simulink model "PMSM_NFLUX_v1_1"  (R2023b)
settings: Solver=FixedStepDiscrete  StartTime=0.0  StopTime=50  FixedStep=0.0001  RelTol=1e-3
values from neighbouring files (symbols this model uses):
  B = 8.0E-5    [PMSM_NFLUX.sldd]    (also in PMSM_NFLUX_backup_before_Simulink_RsStandstillID_20260617_154804.sldd; init_PMSM_NFLUX.m = single(8e-5))
  curr_d_ki = 35.0    [PMSM_NFLUX.sldd]    (also in PMSM_NFLUX_backup_before_Simulink_RsStandstillID_20260617_154804.sldd; init_PMSM_NFLUX.m = 35)
  curr_d_kp = 0.017    [PMSM_NFLUX.sldd]    (also in PMSM_NFLUX_backup_before_Simulink_RsStandstillID_20260617_154804.sldd; init_PMSM_NFLUX.m = 0.017)
  curr_q_ki = 35.0    [PMSM_NFLUX.sldd]    (also in PMSM_NFLUX_backup_before_Simulink_RsStandstillID_20260617_154804.sldd; init_PMSM_NFLUX.m = 35)
  curr_q_kp = 0.017    [PMSM_NFLUX.sldd]    (also in PMSM_NFLUX_backup_before_Simulink_RsStandstillID_20260617_154804.sldd; init_PMSM_NFLUX.m = 0.017)
  flux = 0.016884    [PMSM_NFLUX.sldd]    (also in PMSM_NFLUX_backup_before_Simulink_RsStandstillID_20260617_154804.sldd; init_PMSM_NFLUX.m = single(0.016884))
  Gamma = 100000.0    [PMSM_NFLUX.sldd]    (also in PMSM_NFLUX_backup_before_Simulink_RsStandstillID_20260617_154804.sldd; init_PMSM_NFLUX.m = single(100000.0))
  iq_handover = 0.4    [PMSM_NFLUX.sldd]    (also in PMSM_NFLUX_backup_before_Simulink_RsStandstillID_20260617_154804.sldd; init_PMSM_NFLUX.m = single(0.4))
  iq_ref_slew_down = 2.0    [PMSM_NFLUX.sldd]    (also in PMSM_NFLUX_backup_before_Simulink_RsStandstillID_20260617_154804.sldd; init_PMSM_NFLUX.m = single(2.0))
  iq_ref_slew_up = 5.0    [PMSM_NFLUX.sldd]    (also in PMSM_NFLUX_backup_before_Simulink_RsStandstillID_20260617_154804.sldd; init_PMSM_NFLUX.m = single(5.0))
  J = 7.5E-5    [PMSM_NFLUX.sldd]    (also in PMSM_NFLUX_backup_before_Simulink_RsStandstillID_20260617_154804.sldd; init_PMSM_NFLUX.m = single(75e-6))
  L = 0.00535    [PMSM_NFLUX.sldd]    (also in PMSM_NFLUX_backup_before_Simulink_RsStandstillID_20260617_154804.sldd; init_PMSM_NFLUX.m = single(0.00535))
  load_torque = 0.0    [PMSM_NFLUX.sldd]    (also in PMSM_NFLUX_backup_before_Simulink_RsStandstillID_20260617_154804.sldd; init_PMSM_NFLUX.m = single(0.0))
  LPF_K = 0.003    [PMSM_NFLUX.sldd]    (also in PMSM_NFLUX_backup_before_Simulink_RsStandstillID_20260617_154804.sldd; init_PMSM_NFLUX.m = single(0.003))
  PLL_Ki = 2500.0    [PMSM_NFLUX.sldd]    (also in PMSM_NFLUX_backup_before_Simulink_RsStandstillID_20260617_154804.sldd; init_PMSM_NFLUX.m = single(2500))
  PLL_Kp = 212.1    [PMSM_NFLUX.sldd]    (also in PMSM_NFLUX_backup_before_Simulink_RsStandstillID_20260617_154804.sldd; init_PMSM_NFLUX.m = single(212.1))
  PLL_OmegaLimit = 6283.18555    [PMSM_NFLUX.sldd]    (also in PMSM_NFLUX_backup_before_Simulink_RsStandstillID_20260617_154804.sldd; init_PMSM_NFLUX.m = single(2.0 * pi * 1000.0))
  Pn = 4.0    [PMSM_NFLUX.sldd]    (also in PMSM_NFLUX_backup_before_Simulink_RsStandstillID_20260617_154804.sldd; init_PMSM_NFLUX.m = single(4))
  PWM_HalfPeriod = 8000.0    [PMSM_NFLUX.sldd]    (also in PMSM_NFLUX_backup_before_Simulink_RsStandstillID_20260617_154804.sldd; init_PMSM_NFLUX.m = single(8000))
  Rs = 6.97    [PMSM_NFLUX.sldd]    (also in PMSM_NFLUX_backup_before_Simulink_RsStandstillID_20260617_154804.sldd; init_PMSM_NFLUX.m = single(6.97))
  spd_ki = 0.00165394868    [PMSM_NFLUX.sldd]    (also in PMSM_NFLUX_backup_before_Simulink_RsStandstillID_20260617_154804.sldd; init_PMSM_NFLUX.m = (B * speed_bw / Kt) * rpm_to_radps)
  spd_kp = 0.001550577    [PMSM_NFLUX.sldd]    (also in PMSM_NFLUX_backup_before_Simulink_RsStandstillID_20260617_154804.sldd; init_PMSM_NFLUX.m = (J * speed_bw / Kt) * rpm_to_radps)
  theta_handover_slew_limit = 5.0    [PMSM_NFLUX.sldd]    (also in PMSM_NFLUX_backup_before_Simulink_RsStandstillID_20260617_154804.sldd; init_PMSM_NFLUX.m = single(5.0))
  Tpwm = 16000.0    [PMSM_NFLUX.sldd]    (also in PMSM_NFLUX_backup_before_Simulink_RsStandstillID_20260617_154804.sldd; init_PMSM_NFLUX.m = 2 * PWM_HalfPeriod)
  Ts = 0.0001    [PMSM_NFLUX.sldd]    (also in PMSM_NFLUX_backup_before_Simulink_RsStandstillID_20260617_154804.sldd; init_PMSM_NFLUX.m = 0.0001)
  Udc = 24.0    [PMSM_NFLUX.sldd]    (also in PMSM_NFLUX_backup_before_Simulink_RsStandstillID_20260617_154804.sldd; init_PMSM_NFLUX.m = single(24.0))
undefined symbols (not defined in the file or in its folder): DiscIntNeverNeededParam, magnitude, sigbuilder_block
libraries: slpidlib x4, mcbplantlib x1, simulink x1, autolibpmsmexterior x1
(part 2 of 2)

== system PMSM_NFLUX_v1_1/FOC/current_loop/SVPWM/ei_t ==
  Vabc : Inport  OutDataTypeStr=single
  Demux : Demux  Outputs=3
  Gain : Gain  Gain=-1/2  OutDataTypeStr=single
  Min : MinMax  Inputs=3  OutDataTypeStr=single
  Min1 : MinMax  Function=max  Inputs=3  OutDataTypeStr=single
  Sum : Sum  Inputs=|++  OutDataTypeStr=single
  ei_t : Outport  OutDataTypeStr=single
  wires:
  Min/1 -> Sum/1
  Sum/1 -> Gain/1
  Min1/1 -> Sum/2
  Gain/1 -> ei_t/1
  Vabc/1 -> Demux/1
  Demux/1 -> Min1/1, Min/1
  Demux/2 -> Min/2, Min1/2
  Demux/3 -> Min1/3, Min/3

== system PMSM_NFLUX_v1_1/FOC/current_loop/Subsystem/If Action Subsystem ==
  Action Port : ActionPort  ActionPortLabel=case [ 1 ]:
  Constant : Constant  Value=0  OutDataTypeStr=single
  Constant1 : Constant  Value=0  OutDataTypeStr=single
  theta_fd : Outport
  iq_ref : Outport  Port=2
  wires:
  Constant/1 -> theta_fd/1
  Constant1/1 -> iq_ref/1

== system PMSM_NFLUX_v1_1/FOC/current_loop/Subsystem/If Action Subsystem1 ==
  Action Port : ActionPort  ActionPortLabel=case [ 2 ]:
  Constant : Constant  Value=0  OutDataTypeStr=single
  Constant1 : Constant  OutDataTypeStr=single
  theta_fd : Outport
  iq_ref : Outport  Port=2
  wires:
  Constant1/1 -> iq_ref/1
  Constant/1 -> theta_fd/1

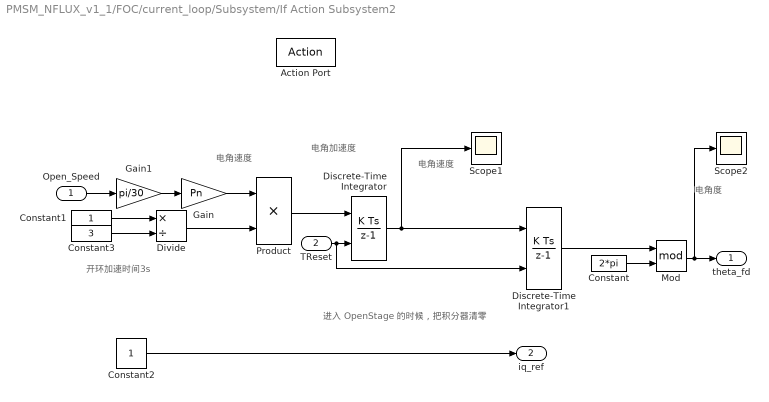
== system PMSM_NFLUX_v1_1/FOC/current_loop/Subsystem/If Action Subsystem2 ==
  note: 进入 OpenStage 的时候，把积分器清零
  note: 电角速度
  note: 开环加速时间3s
  note: 电角加速度
  note: 电角速度
  note: 电角度
  Open_Speed : Inport  OutDataTypeStr=int32  PortDimensions=1
  TReset : Inport  Port=2
  Action Port : ActionPort  ActionPortLabel=case [ 3 ]:
  Constant : Constant  Value=2*pi  OutDataTypeStr=single
  Constant1 : Constant  OutDataTypeStr=single
  Constant2 : Constant  OutDataTypeStr=single
  Constant3 : Constant  Value=3  OutDataTypeStr=single
  Discrete-Time Integrator : DiscreteIntegrator  ExternalReset=rising  SampleTime=-1  ICPrevOutput=DiscIntNeverNeededParam  ICPrevScaledInput=DiscIntNeverNeededParam
  Discrete-Time Integrator1 : DiscreteIntegrator  ExternalReset=rising  SampleTime=-1  ICPrevOutput=DiscIntNeverNeededParam  ICPrevScaledInput=DiscIntNeverNeededParam
  Divide : Product  Inputs=*/  OutDataTypeStr=single
  Gain : Gain  Gain=Pn
  Gain1 : Gain  Gain=pi/30  OutDataTypeStr=single
  Mod : Math  Operator=mod
  Product : Product  OutDataTypeStr=single
  Scope1 : Scope
  Scope2 : Scope
  theta_fd : Outport
  iq_ref : Outport  Port=2
  wires:
  Gain1/1 -> Gain/1
  Constant1/1 -> Divide/1
  Gain/1 -> Product/1
  Constant/1 -> Mod/2
  Discrete-Time Integrator1/1 -> Mod/1
  Mod/1 -> Scope2/1, theta_fd/1
  Constant3/1 -> Divide/2
  Constant2/1 -> iq_ref/1
  Divide/1 -> Product/2
  Product/1 -> Discrete-Time Integrator/1
  Open_Speed/1 -> Gain1/1
  TReset/1 -> Discrete-Time Integrator1/2, Discrete-Time Integrator/2
  Discrete-Time Integrator/1 -> Scope1/1, Discrete-Time Integrator1/1

== system PMSM_NFLUX_v1_1/FOC/current_loop/Subsystem/If Action Subsystem3 ==
  theta_Close : Inport
  iq_CloseRef : Inport  Port=2
  Action Port : ActionPort  ActionPortLabel=case [ 5 ]:
  theta_fd : Outport
  iq_ref : Outport  Port=2
  wires:
  theta_Close/1 -> theta_fd/1
  iq_CloseRef/1 -> iq_ref/1

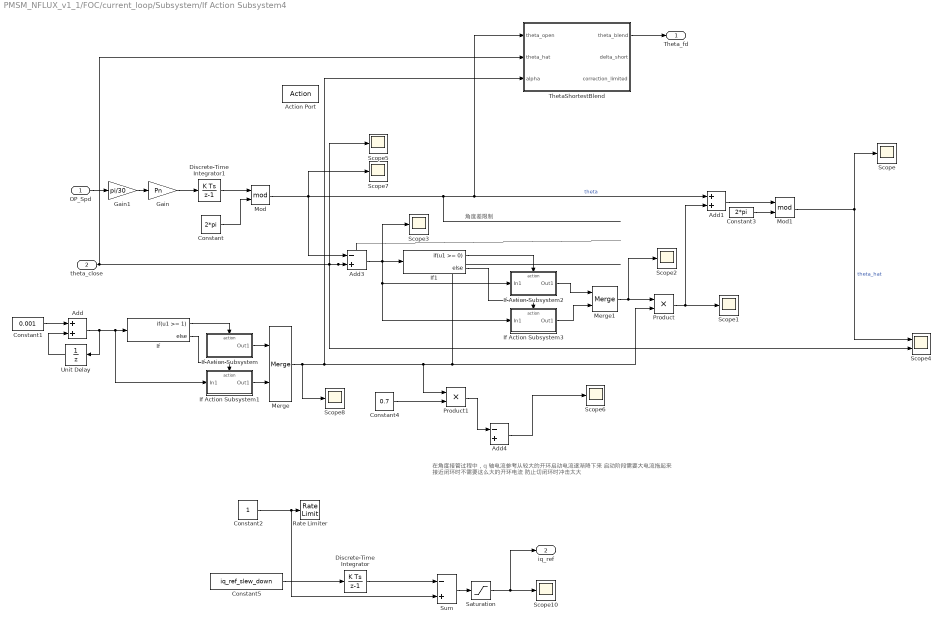
== system PMSM_NFLUX_v1_1/FOC/current_loop/Subsystem/If Action Subsystem4 ==
  note: 在角度接管过程中，q 轴电流参考从较大的开环启动电流逐渐降下来
      | 启动阶段需要大电流拖起来
      | 接近闭环时不需要这么大的开环电流
      | 防止切闭环时冲击太大
  note: 角度差限制
  OP_Spd : Inport  OutDataTypeStr=int32  PortDimensions=1
  theta_close : Inport  Port=2
  Action Port : ActionPort  ActionPortLabel=case [ 4 ]:
  Add : Sum
  Add1 : Sum
  Add3 : Sum  Inputs=-+
  Add4 : Sum  Inputs=-+
  Constant : Constant  Value=2*pi  OutDataTypeStr=single
  Constant1 : Constant  Value=0.001  OutDataTypeStr=single
  Constant2 : Constant  OutDataTypeStr=single
  Constant3 : Constant  Value=2*pi  OutDataTypeStr=single
  Constant4 : Constant  Value=0.7  OutDataTypeStr=single
  Constant5 : Constant  Value=iq_ref_slew_down
  Discrete-Time Integrator : DiscreteIntegrator  SampleTime=-1  ICPrevOutput=DiscIntNeverNeededParam  ICPrevScaledInput=DiscIntNeverNeededParam
  Discrete-Time Integrator1 : DiscreteIntegrator  SampleTime=-1  ICPrevOutput=DiscIntNeverNeededParam  ICPrevScaledInput=DiscIntNeverNeededParam
  Gain : Gain  Gain=Pn
  Gain1 : Gain  Gain=pi/30  OutDataTypeStr=single
  If : If  IfExpression=u1 >= 1
  If Action Subsystem : Subsystem  TreatAsAtomicUnit=on
  If Action Subsystem1 : Subsystem  TreatAsAtomicUnit=on
  If Action Subsystem2 : Subsystem  TreatAsAtomicUnit=on
  If Action Subsystem3 : Subsystem  TreatAsAtomicUnit=on
  If1 : If  IfExpression=u1 >= 0
  Merge : Merge
  Merge1 : Merge
  Mod : Math  Operator=mod
  Mod1 : Math  Operator=mod
  Product : Product
  Product1 : Product
  Rate Limiter : RateLimiter  RisingSlewLimit=iq_ref_slew_up  FallingSlewLimit=-iq_ref_slew_down  SampleTimeMode=inherited  InitialCondition=01
  Saturation : Saturate  UpperLimit=1  LowerLimit=iq_handover
  Scope{,1..3,5..8,10} (9 alike) : Scope
  Scope4 : Scope  NumInputPorts=2
  Sum : Sum  Inputs=-+
  ThetaShortestBlend : Subsystem  TreatAsAtomicUnit=on
  Unit Delay : UnitDelay  SampleTime=-1  HasFrameUpgradeWarning=on
  Theta_fd : Outport
  iq_ref : Outport  Port=2
  wires:
  Gain/1 -> Discrete-Time Integrator1/1
  Constant/1 -> Mod/2
  Discrete-Time Integrator1/1 -> Mod/1
  Constant1/1 -> Add/1
  OP_Spd/1 -> Gain1/1
  If/1 -> If Action Subsystem/Action
  Gain1/1 -> Gain/1
  If Action Subsystem1/1(Out1) -> Merge/2
  Unit Delay/1 -> Add/2
  Add/1 -> Unit Delay/1, If/1, If Action Subsystem1/1(In1)
  If Action Subsystem/1(Out1) -> Merge/1
  If/2 -> If Action Subsystem1/Action
  Add3/1 -> Scope3/1, If Action Subsystem3/1(In1), If Action Subsystem2/1(In1), If1/1
  If1/1 -> If Action Subsystem2/Action
  If1/2 -> If Action Subsystem3/Action
  If Action Subsystem2/1(Out1) -> Merge1/1
  If Action Subsystem3/1(Out1) -> Merge1/2
  Merge1/1 -> Scope2/1, Product/1
  Merge/1 -> ThetaShortestBlend/3(alpha), Product/2, Product1/1, Scope8/1
  Product/1 -> Scope1/1, Add1/2
  Constant3/1 -> Mod1/2
  Add1/1 -> Mod1/1
  Constant4/1 -> Product1/2
  Add4/1 -> Scope6/1
  Mod1/1 -> Scope/1, Scope4/1  "theta_hat"
  Mod/1 -> ThetaShortestBlend/1(theta_open), Add1/1, Scope7/1, Add3/1  "theta"
  theta_close/1 -> Add3/2, Scope4/2, Scope5/1, ThetaShortestBlend/2(theta_hat)
  Product1/1 -> Add4/1
  Constant2/1 -> Sum/2, Rate Limiter/1
  Discrete-Time Integrator/1 -> Sum/1
  Constant5/1 -> Discrete-Time Integrator/1
  Sum/1 -> Saturation/1
  Saturation/1 -> iq_ref/1, Scope10/1
  ThetaShortestBlend/1(theta_blend) -> Theta_fd/1

== system PMSM_NFLUX_v1_1/FOC/current_loop/Subsystem/If Action Subsystem4/If Action Subsystem ==
  Action Port : ActionPort  ActionPortLabel=if(u1 >= 1)
  Constant : Constant  OutDataTypeStr=single
  Out1 : Outport
  wires:
  Constant/1 -> Out1/1

== system PMSM_NFLUX_v1_1/FOC/current_loop/Subsystem/If Action Subsystem4/If Action Subsystem1 ==
  In1 : Inport
  Action Port : ActionPort  ActionPortLabel=else
  Out1 : Outport
  wires:
  In1/1 -> Out1/1

== system PMSM_NFLUX_v1_1/FOC/current_loop/Subsystem/If Action Subsystem4/If Action Subsystem2 ==
  In1 : Inport
  Action Port : ActionPort  ActionPortLabel=if(u1 >= 0)
  Out1 : Outport
  wires:
  In1/1 -> Out1/1

== system PMSM_NFLUX_v1_1/FOC/current_loop/Subsystem/If Action Subsystem4/If Action Subsystem3 ==
  In1 : Inport
  Action Port : ActionPort  ActionPortLabel=else
  Add : Sum
  Constant : Constant  Value=2*pi  OutDataTypeStr=single
  Out1 : Outport
  wires:
  In1/1 -> Add/1
  Constant/1 -> Add/2
  Add/1 -> Out1/1

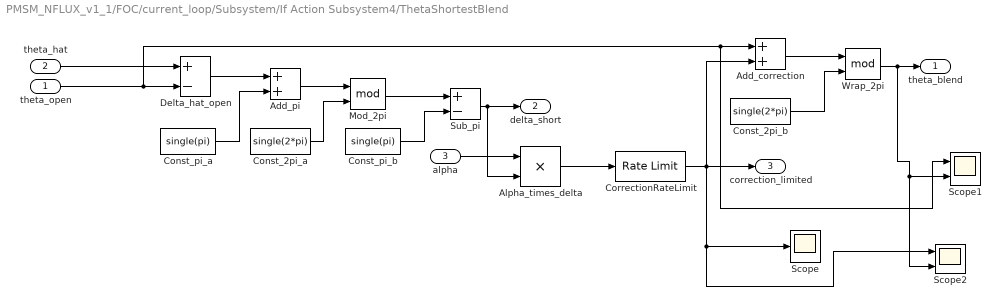
== system PMSM_NFLUX_v1_1/FOC/current_loop/Subsystem/If Action Subsystem4/ThetaShortestBlend ==
  theta_open : Inport
  theta_hat : Inport  Port=2
  alpha : Inport  Port=3
  Add_correction : Sum
  Add_pi : Sum
  Alpha_times_delta : Product
  Const_2pi_a : Constant  Value=single(2*pi)  OutDataTypeStr=single
  Const_2pi_b : Constant  Value=single(2*pi)  OutDataTypeStr=single
  Const_pi_a : Constant  Value=single(pi)  OutDataTypeStr=single
  Const_pi_b : Constant  Value=single(pi)  OutDataTypeStr=single
  CorrectionRateLimit : RateLimiter  RisingSlewLimit=theta_handover_slew_limit  FallingSlewLimit=-theta_handover_slew_limit  SampleTimeMode=inherited
  Delta_hat_open : Sum  Inputs=+-
  Mod_2pi : Math  Operator=mod
  Scope : Scope
  Scope1 : Scope  NumInputPorts=2
  Scope2 : Scope  NumInputPorts=2
  Sub_pi : Sum  Inputs=+-
  Wrap_2pi : Math  Operator=mod
  theta_blend : Outport
  delta_short : Outport  Port=2
  correction_limited : Outport  Port=3
  wires:
  Mod_2pi/1 -> Sub_pi/1
  Add_pi/1 -> Mod_2pi/1
  theta_hat/1 -> Delta_hat_open/1
  Sub_pi/1 -> Alpha_times_delta/2, delta_short/1
  theta_open/1 -> Scope1/1, Add_correction/1, Delta_hat_open/2
  Delta_hat_open/1 -> Add_pi/1
  alpha/1 -> Alpha_times_delta/1
  Const_pi_a/1 -> Add_pi/2
  Const_2pi_b/1 -> Wrap_2pi/2
  Const_pi_b/1 -> Sub_pi/2
  Const_2pi_a/1 -> Mod_2pi/2
  Alpha_times_delta/1 -> CorrectionRateLimit/1
  Add_correction/1 -> Wrap_2pi/1
  CorrectionRateLimit/1 -> Scope2/1, Scope/1, Add_correction/2, correction_limited/1
  Wrap_2pi/1 -> Scope2/2, Scope1/2, theta_blend/1

== matlab function PMSM_NFLUX_v1_1/FOC/current_loop/SVPWM/MATLAB Function ==
  data: Ualpha input; T1 output; Ubeta input; Udc input; Tpwm input; T2 output; T3 output; sector output
function [T1,T2,T3,sector] = fcn(Ualpha,Ubeta,Udc,Tpwm)

% 初始化
sector = single(0);
T1 = single(0);
T2 = single(0);
T3 = single(0);

% 第一步：扇区判断
% 计算三个临时变量
Ua = Ubeta;
Ub = (sqrt(3)*Ualpha - Ubeta)/2;
Uc = (-sqrt(3)*Ualpha - Ubeta)/2;
% 计算判断扇区所用的ABC的值
A=single(0);B=single(0);C=single(0);N=single(0);
if(Ua>0)
    A = single(1);
elseif(Ua<0)
    A = single(0);
end
if(Ub>0)
    B = single(1);
elseif(Ub<0)
    B = single(0);
end
if(Uc>0)
    C = single(1);
elseif(Uc<0)
    C = single(0);
end
% 计算判断扇区所用的N的值
N = A + 2*B + 4*C;
% 扇区判断
switch (N)   
    case 3
        sector = single(1);
    case 1
        sector = single(2);
    case 5
        sector = single(3);
    case 4
        sector = single(4);
    case 6
        sector = single(5);
    case 2
        sector = single(6);
end

% 第二步：计算相邻矢量作用时长
% 计算调制比
Umr = sqrt(3)*Tpwm/Udc;
% 计算三个临时变量
X = Umr * Ua;
Y = Umr * Ub;
Z = Umr * Uc;
% 分扇区计算Tx和Ty的值
Tx=single(0);Ty=single(0);
switch (sector)
    case 1
        Tx = Y; Ty = X;
    case 2
        Tx = -Y; Ty = -Z;
    case 3
        Tx = X; Ty = Z;
    case 4
        Tx = -X; Ty = -Y;
    case 5
        Tx = Z; Ty = Y;
    case 6
        Tx = -Z; Ty = -X;
end

% 第三步：定时器比较值计算
% 干啥用的？
if Tx+Ty > Tpwm
    Tx = Tx/(Tx+Ty);
    Ty = Ty/(Tx+Ty);
else
    Tx = Tx;
    Ty = Ty;
end
% 计算三个临时变量
Ta = (Tpwm-Tx-Ty)/4.0;
Tb = Ta+Tx/2.0;
Tc = Tb+Ty/2.0;
% 分扇区计算定时器比较值T1、T2和T3的值
switch (sector)
    case 1
        T1 = Ta; T2 = Tb; T3 = Tc;
    case 2
        T1 = Tb; T2 = Ta; T3 = Tc;
    case 3
        T1 = Tc; T2 = Ta; T3 = Tb;
    case 4
        T1 = Tc; T2 = Tb; T3 = Ta;
    case 5
        T1 = Tb; T2 = Tc; T3 = Ta;
    case 6
        T1 = Ta; T2 = Tc; T3 = Tb;
end

end

== stateflow chart PMSM_NFLUX_v1_1/FOC/current_loop/Subsystem/Chart ==
  note: %after表示Stateflow执行了多少次
  state OpenStage%开环爬升，ZRset,cnt初始化
    en:
    cnt = 0;
    du:
    Motor_state = 3;
    RestsSingal = 0;
    if cnt == 0
    ZReset = 1;
    cnt = 1;
    else
    ZReset = 0;
    end
  state ThetaAlign%角度接管/偏差校正
    %准备从开环角度过渡到观测器角度
    en:
    du:
    ZReset = 0;
    Motor_state = 4;
    RestsSingal = 0;
  state IDLE
    en:
    du:
    ZReset = 0;
    Motor_state = 1;
    RestsSingal = 0;
  state RunStage%正式闭环运行
    en:
    du:
    ZReset = 0;
    Motor_state = 5;
    RestsSingal = 1;
  state AlignStage%对齐转子
    en:
    du:
    ZReset = 0;
    Motor_state = 2;
    RestsSingal = 0;
  (default) -> IDLE
  ThetaAlign%角度接管/偏差校正 -> RunStage%正式闭环运行 [order 1] : [after(5000,tick)]
  IDLE -> AlignStage%对齐转子 : [Motor_OnOff == 1]
  AlignStage%对齐转子 -> OpenStage%开环爬升，ZRset,cnt初始化 [order 1] : [after(1000,tick)]
  OpenStage%开环爬升，ZRset,cnt初始化 -> ThetaAlign%角度接管/偏差校正 [order 1] : [after(30000,tick)&&OpenLoopHold == 0]
  AlignStage%对齐转子 -> IDLE [order 2] : [Motor_OnOff == 0]
  ThetaAlign%角度接管/偏差校正 -> IDLE [order 2] : [Motor_OnOff == 0]
  OpenStage%开环爬升，ZRset,cnt初始化 -> IDLE [order 2] : [Motor_OnOff == 0]
  RunStage%正式闭环运行 -> IDLE : [Motor_OnOff == 0]
  data: Motor_OnOff input; OpenLoopHold input; Motor_state output; RestsSingal output; ZReset output; cnt local
